simulink model "Model_lab3"  (R2020a)
settings: Solver=ode1  StartTime=0.0  StopTime=simul_t  RelTol=1e-3
values from neighbouring files (symbols this model uses):
  Kp = Kd    [script_lab3.m]
  Kt = 3.575*10^(-5)    (= 3.575e-05)    [script_lab3.m]
  M = 1    [script_lab3.m]
  Omega_0 = sqrt((G*M)/Kt)    [script_lab3.m]
undefined symbols (not defined in the file or in its folder): dz_r
settings Model: Creator=lucas  LastModifiedBy=lucas

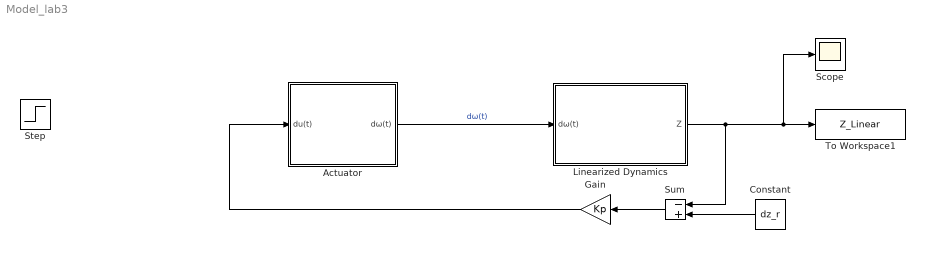
== system Model_lab3 ==
  Actuator : Subsystem
  Constant : Constant  Value=dz_r
  Gain : Gain  Gain=Kp
  Linearized Dynamics : Subsystem
  Scope : Scope
  Step : Step  SampleTime=0
  Sum : Sum  Inputs=-+
  To Workspace1 : ToWorkspace  VariableName=Z_Linear  SaveFormat=Structure With Time  SampleTime=-1
  wires:
  Linearized Dynamics/1(Z) -> Scope/1, To Workspace1/1, Sum/1
  Actuator/1(dω(t)) -> Linearized Dynamics/1(dω(t))  "dω(t)"
  Constant/1 -> Sum/2
  Sum/1 -> Gain/1
  Gain/1 -> Actuator/1(du(t))

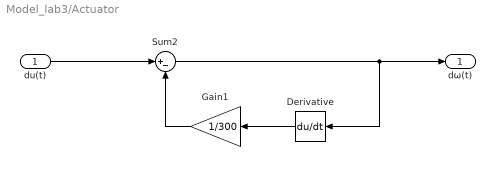
== system Model_lab3/Actuator ==
  du(t) : Inport
  Derivative : Derivative
  Gain1 : Gain  Gain=1/300
  Sum2 : Sum  Inputs=|+-
  dω(t) : Outport
  wires:
  du(t)/1 -> Sum2/1
  Sum2/1 -> dω(t)/1, Derivative/1
  Derivative/1 -> Gain1/1
  Gain1/1 -> Sum2/2

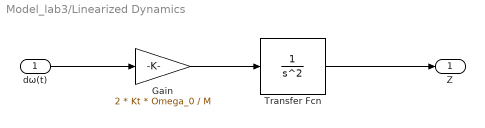
== system Model_lab3/Linearized Dynamics ==
  dω(t) : Inport
  Gain : Gain  Gain=2 * Kt * Omega_0 / M
  Transfer Fcn : TransferFcn  Denominator=[1 0 0]
  Z : Outport
  wires:
  dω(t)/1 -> Gain/1
  Gain/1 -> Transfer Fcn/1
  Transfer Fcn/1 -> Z/1
